simulink subsystem "DCmotor"  (R2023a)
settings: Solver=VariableStepAuto  StartTime=0.0  StopTime=10.0  RelTol=1e-3
model mask{Pn=0, Nn=0, Un=0, In=0, Ra=0, Im=0}
  mask prompts: Pn "Номинальная мощность, Вт"; Nn "Номинальная частота вращения, об/мин"; Un "Номинальное напряжение питания, В"; In "Номинальный ток якоря, А"; Ra "Сопротивление обмотки якоря, Ом"; Im "Момент инерции двигателя, кг*м^2"
undefined symbols (not defined in the file): Km, Kw, Te
settings Model: Creator=user  LastModifiedBy=user

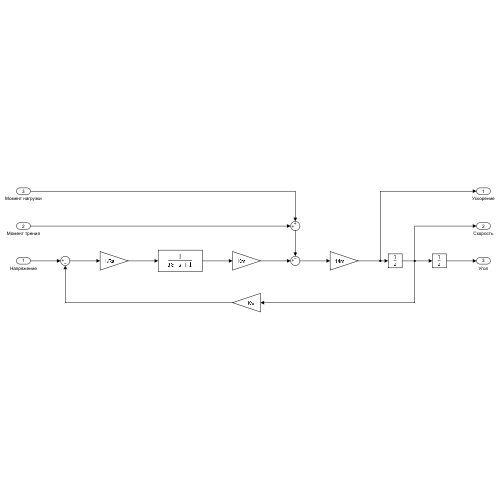
[thumbnail: Simulink's stored preview of the top-level diagram]
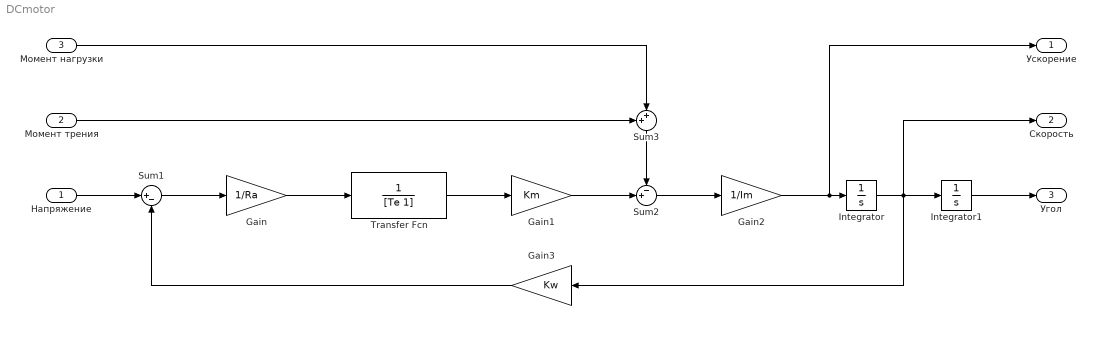
== system DCmotor ==
  Напряжение : Inport
  Момент трения : Inport  Port=2
  Момент нагрузки : Inport  Port=3
  Gain : Gain  Gain=1/Ra
  Gain1 : Gain  Gain=Km
  Gain2 : Gain  Gain=1/Im
  Gain3 : Gain  Gain=Kw
  Integrator : Integrator
  Integrator1 : Integrator
  Sum1 : Sum  Inputs=|+-
  Sum2 : Sum  Inputs=-+|
  Sum3 : Sum  Inputs=++|
  Transfer Fcn : TransferFcn  Denominator=[Te 1]
  Ускорение : Outport
  Скорость : Outport  Port=2
  Угол : Outport  Port=3
  wires:
  Integrator1/1 -> Угол/1
  Момент трения/1 -> Sum3/1
  Момент нагрузки/1 -> Sum3/2
  Gain/1 -> Transfer Fcn/1
  Gain1/1 -> Sum2/2
  Напряжение/1 -> Sum1/1
  Gain2/1 -> Ускорение/1, Integrator/1
  Sum2/1 -> Gain2/1
  Integrator/1 -> Скорость/1, Gain3/1, Integrator1/1
  Gain3/1 -> Sum1/2
  Transfer Fcn/1 -> Gain1/1
  Sum1/1 -> Gain/1
  Sum3/1 -> Sum2/1
